simulink model "Ex_Solve_DiffEqn_Simulink"  (R2018a)
settings: Solver=FixedStepAuto  StartTime=0.0  StopTime=t(end)  FixedStep=Ts  RelTol=1e-3
values from neighbouring files (symbols this model uses):
  B = 10    [Part3_Solve_Sys_LinearNL_Eqn_DiffEqn.m]    (also in Part3_Solve_Sys_LinearNL_Eqn_DiffEqn_Template.m; diff_eqn_1.m = params.B)
  K = 100    [Part3_Solve_Sys_LinearNL_Eqn_DiffEqn.m]    (also in Part3_Solve_Sys_LinearNL_Eqn_DiffEqn_Template.m; diff_eqn_1.m = params.K)
  M = 10    [Part3_Solve_Sys_LinearNL_Eqn_DiffEqn.m]    (also in Part3_Solve_Sys_LinearNL_Eqn_DiffEqn_Template.m; diff_eqn_1.m = params.M)
  Ts = 10^-3    (= 0.001)    [Part3_Solve_Sys_LinearNL_Eqn_DiffEqn.m]    (also in Part3_Solve_Sys_LinearNL_Eqn_DiffEqn_Template.m)
settings Model: Creator=strikefreedom2017  LastModifiedBy=strikefreedom2017

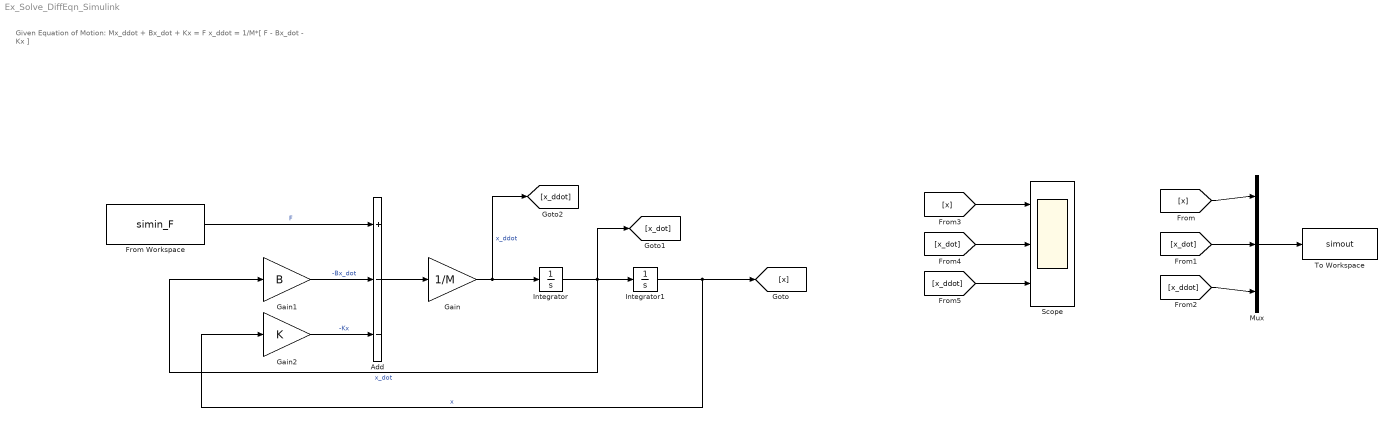
== system Ex_Solve_DiffEqn_Simulink ==
  note: Given Equation of Motion:
      | Mx_ddot + Bx_dot + Kx = F
      |
      | x_ddot = 1/M*[ F - Bx_dot - Kx ]
  Add : Sum  Inputs=+--
  From Workspace : FromWorkspace  VariableName=simin_F  SampleTime=Ts
  Gain : Gain  Gain=1/M
  Gain1 : Gain  Gain=B
  Gain2 : Gain  Gain=K
  Integrator : Integrator
  Integrator1 : Integrator
  Mux : Mux  Inputs=3
  Scope : Scope  NumInputPorts=3
  To Workspace : ToWorkspace  VariableName=simout  SaveFormat=Timeseries  SampleTime=-1
  wires:
  Add/1 -> Gain/1
  Gain1/1 -> Add/2  "-Bx_dot"
  Gain2/1 -> Add/3  "-Kx"
  Gain/1 -> [x_ddot], Integrator/1  "x_ddot"
  Integrator/1 -> [x_dot], Gain1/1, Integrator1/1  "x_dot"
  Integrator1/1 -> [x], Gain2/1  "x"
  From Workspace/1 -> Add/1  "F"
  [x] -> Mux/1
  [x_dot] -> Mux/2
  [x_ddot] -> Mux/3
  Mux/1 -> To Workspace/1
  [x] -> Scope/1
  [x_ddot] -> Scope/3
  [x_dot] -> Scope/2
